simulink model "mc_pos"  (R2021a)
settings: Solver=FixedStepAuto  StartTime=0.0  StopTime=10.0  FixedStep=0.1  RelTol=1e-3
undefined symbols (not defined in the file): CONSTANTS_ONE_G, DiscIntNeverNeededParam, MPC_LAND_SPEED, MPC_SPOOLUP_TIME, MPC_THR_HOVER, MPC_THR_MAX, MPC_THR_MIN, MPC_TILTMAX_AIR, MPC_TILTMAX_LND, MPC_TKO_RAMP_T, MPC_VELD_LP, MPC_XY_P, MPC_XY_VEL_D_ACC, MPC_XY_VEL_I_ACC, MPC_XY_VEL_MAX, MPC_XY_VEL_P_ACC, MPC_Z_P, MPC_Z_VEL_D_ACC, MPC_Z_VEL_I_ACC, MPC_Z_VEL_MAX_DN, MPC_Z_VEL_MAX_UP, MPC_Z_VEL_P_ACC, PX4_TAKEOFF_STATUS, WV_EN
libraries: simulink x16, vrlib x2, sharedtransform x2, aerolibconvert2 x1
(part 2 of 3)

== system mc_pos/Position Controller/Position Control/addIfNotNan ==
  setpoint : Inport
  addition : Inport  Port=2
  AND : Logic  AllPortsSameDT=off  OutDataTypeStr=boolean
  IsFinite : RelationalOperator  Operator=isFinite  OutDataTypeStr=boolean  RndMeth=Simplest
  IsFinite1 : RelationalOperator  Operator=isFinite  OutDataTypeStr=boolean  RndMeth=Simplest
  IsFinite3 : RelationalOperator  Operator=isFinite  OutDataTypeStr=boolean  RndMeth=Simplest
  Sum : Sum  Inputs=++|
  Switch : Switch  Criteria=u2 ~= 0
  Switch1 : Switch  Criteria=u2 ~= 0
  addition1 : InportShadow  Port=2
  addition2 : InportShadow  Port=2
  setpoint1 : InportShadow
  setpoint2 : InportShadow
  sp_out : Outport
  wires:
  setpoint/1 -> IsFinite/1
  addition/1 -> IsFinite1/1
  IsFinite/1 -> AND/1
  IsFinite1/1 -> AND/2
  AND/1 -> Switch/2
  Sum/1 -> Switch/1
  setpoint1/1 -> Sum/2
  addition1/1 -> Sum/1
  Switch1/1 -> Switch/3
  setpoint2/1 -> IsFinite3/1, Switch1/1
  IsFinite3/1 -> Switch1/2
  addition2/1 -> Switch1/3
  Switch/1 -> sp_out/1

== system mc_pos/Position Controller/Position Control/addIfNotNan1 ==
  setpoint : Inport
  addition : Inport  Port=2
  AND : Logic  AllPortsSameDT=off  OutDataTypeStr=boolean
  IsFinite : RelationalOperator  Operator=isFinite  OutDataTypeStr=boolean  RndMeth=Simplest
  IsFinite1 : RelationalOperator  Operator=isFinite  OutDataTypeStr=boolean  RndMeth=Simplest
  IsFinite3 : RelationalOperator  Operator=isFinite  OutDataTypeStr=boolean  RndMeth=Simplest
  Sum : Sum  Inputs=++|
  Switch : Switch  Criteria=u2 ~= 0
  Switch1 : Switch  Criteria=u2 ~= 0
  addition1 : InportShadow  Port=2
  addition2 : InportShadow  Port=2
  setpoint1 : InportShadow
  setpoint2 : InportShadow
  sp_out : Outport
  wires:
  Switch/1 -> sp_out/1
  addition2/1 -> Switch1/3
  IsFinite3/1 -> Switch1/2
  setpoint2/1 -> Switch1/1, IsFinite3/1
  Switch1/1 -> Switch/3
  addition1/1 -> Sum/1
  setpoint1/1 -> Sum/2
  Sum/1 -> Switch/1
  AND/1 -> Switch/2
  IsFinite1/1 -> AND/2
  IsFinite/1 -> AND/1
  addition/1 -> IsFinite1/1
  setpoint/1 -> IsFinite/1

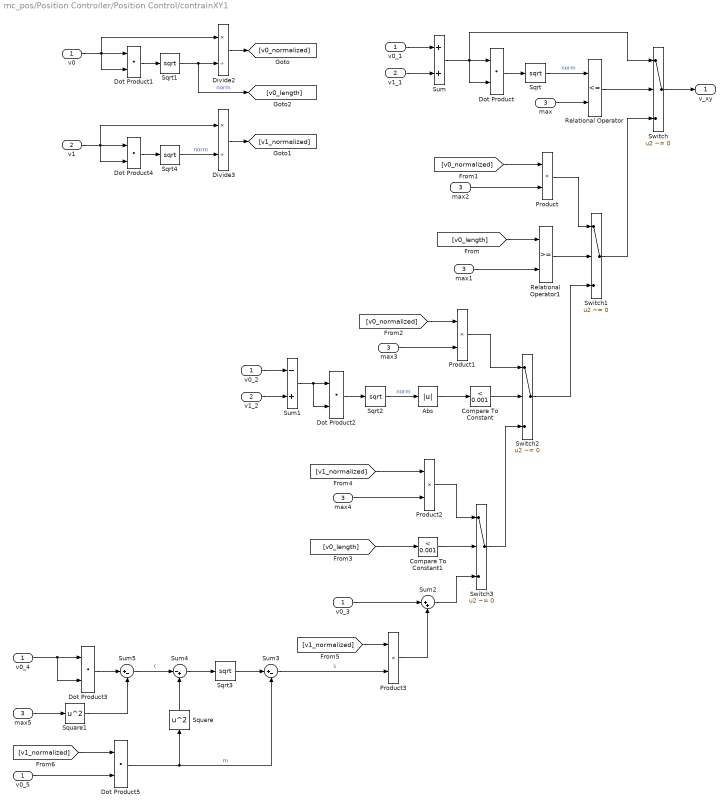
== system mc_pos/Position Controller/Position Control/contrainXY1 ==
  v0 : Inport
  v1 : Inport  Port=2
  max : Inport  Port=3
  Abs : Abs
  Compare To Constant : simulink/Logic and Bit Operations/Compare To Constant  relop=<  const=0.001  OutDataTypeStr=boolean
  Compare To Constant1 : simulink/Logic and Bit Operations/Compare To Constant  relop=<  const=0.001  OutDataTypeStr=boolean
  Divide2 : Product  Inputs=*/
  Divide3 : Product  Inputs=*/
  Dot Product{,1..5} (6 alike) : DotProduct  InputSameDT=on  OutDataTypeStr=Inherit: Inherit via internal rule
  Product{,1..3} (4 alike) : Product
  Relational Operator : RelationalOperator  Operator=<=  OutDataTypeStr=boolean  RndMeth=Simplest
  Relational Operator1 : RelationalOperator  OutDataTypeStr=boolean  RndMeth=Simplest
  Sqrt{,1..4} (5 alike) : Sqrt  SaturateOnIntegerOverflow=on
  Square : Math  Operator=square  SaturateOnIntegerOverflow=on
  Square1 : Math  Operator=square  SaturateOnIntegerOverflow=on
  Sum : Sum
  Sum1 : Sum  Inputs=-+
  Sum2 : Sum  Inputs=|++
  Sum3 : Sum  Inputs=|+-
  Sum4 : Sum  Inputs=|-+
  Sum5 : Sum  Inputs=|+-
  Switch{,1..3} (4 alike) : Switch  Criteria=u2 ~= 0
  max{1..5} (5 alike) : InportShadow  Port=3
  v0_{1..5} (5 alike) : InportShadow
  v1_1 : InportShadow  Port=2
  v1_2 : InportShadow  Port=2
  v_xy : Outport
  wires:
  v0_5/1 -> Dot Product5/2
  [v1_normalized] -> Dot Product5/1
  Square1/1 -> Sum5/2
  max5/1 -> Square1/1
  Dot Product3/1 -> Sum5/1
  v0_4/1 -> Dot Product3/1, Dot Product3/2
  Sum5/1 -> Sum4/1  "c"
  Square/1 -> Sum4/2
  Dot Product5/1 -> Sum3/2, Square/1  "m"
  Sum4/1 -> Sqrt3/1
  Sqrt3/1 -> Sum3/1
  Sum3/1 -> Product3/2  "s"
  [v1_normalized] -> Product3/1
  Product3/1 -> Sum2/2
  v0_3/1 -> Sum2/1
  Sum2/1 -> Switch3/3
  [v1_normalized] -> Product2/1
  max4/1 -> Product2/2
  Product2/1 -> Switch3/1
  [v0_length] -> Compare To Constant1/1
  Compare To Constant1/1 -> Switch3/2
  max3/1 -> Product1/2
  Product1/1 -> Switch2/1
  [v0_normalized] -> Product/1
  [v0_length] -> Relational Operator1/1
  Divide3/1 -> [v1_normalized]
  v1/1 -> Dot Product4/1, Dot Product4/2, Divide3/1
  Dot Product4/1 -> Sqrt4/1
  Sqrt4/1 -> Divide3/2  "norm"
  Divide2/1 -> [v0_normalized]
  Switch3/1 -> Switch2/3
  [v0_normalized] -> Product1/1
  v0_2/1 -> Sum1/1
  v1_2/1 -> Sum1/2
  Compare To Constant/1 -> Switch2/2
  Abs/1 -> Compare To Constant/1
  Sqrt2/1 -> Abs/1  "norm"
  Dot Product2/1 -> Sqrt2/1
  Sum1/1 -> Dot Product2/1, Dot Product2/2
  Switch2/1 -> Switch1/3
  Product/1 -> Switch1/1
  max2/1 -> Product/2
  Relational Operator1/1 -> Switch1/2
  max1/1 -> Relational Operator1/2
  Sqrt1/1 -> Divide2/2, [v0_length]  "norm"
  Dot Product1/1 -> Sqrt1/1
  v0/1 -> Dot Product1/1, Divide2/1, Dot Product1/2
  Switch1/1 -> Switch/3
  Switch/1 -> v_xy/1
  Relational Operator/1 -> Switch/2
  max/1 -> Relational Operator/2
  Sqrt/1 -> Relational Operator/1  "norm"
  Dot Product/1 -> Sqrt/1
  Sum/1 -> Dot Product/1, Dot Product/2, Switch/1
  v0_1/1 -> Sum/1
  v1_1/1 -> Sum/2

== system mc_pos/Position Controller/Velocity Control/I ==
  vel_error : Inport
  acc_sp : Inport  Port=2
  last_thr_sp : Inport  Port=3
  Bus Element In : Inport  Port=4  PortName=limit
  reset : Inport  Port=5
  Anti-Windup Calculate Velocity Error : Subsystem
  Constant : Constant  Value=[0 0 0]  OutDataTypeStr=single
  Discrete-Time Integrator : DiscreteIntegrator  ExternalReset=level  SampleTime=-1  SaturateOnIntegerOverflow=on  LimitOutput=on  UpperSaturationLimit=[inf inf CONSTANTS_ONE_G]  LowerSaturationLimit=-[inf inf CONSTANTS_ONE_G]  ICPrevOutput=DiscIntNeverNeededParam  ICPrevScaledInput=DiscIntNeverNeededParam
  Gain : Gain  Gain=[MPC_XY_VEL_I_ACC; MPC_XY_VEL_I_ACC; MPC_Z_VEL_I_ACC]
      settings: AttributesFormatString=%<Gain>
  addIfNotNan : Subsystem
  vel_init : Outport
  wires:
  Gain/1 -> Discrete-Time Integrator/1
  last_thr_sp/1 -> Anti-Windup Calculate Velocity Error/3(last_thr_sp)
  Bus Element In/1 -> Anti-Windup Calculate Velocity Error/4(limit)
  vel_error/1 -> Anti-Windup Calculate Velocity Error/1(vel_error)
  acc_sp/1 -> Anti-Windup Calculate Velocity Error/2(acc_sp)
  Discrete-Time Integrator/1 -> vel_init/1
  reset/1 -> Discrete-Time Integrator/2
  Anti-Windup Calculate Velocity Error/1(vel_error_out) -> addIfNotNan/1(setpoint)
  Constant/1 -> addIfNotNan/2(addition)
  addIfNotNan/1(sp_out) -> Gain/1

== system mc_pos/Position Controller/Velocity Control/addIfNotNan ==
  setpoint : Inport
  addition : Inport  Port=2
  AND : Logic  AllPortsSameDT=off  OutDataTypeStr=boolean
  IsFinite : RelationalOperator  Operator=isFinite  OutDataTypeStr=boolean  RndMeth=Simplest
  IsFinite1 : RelationalOperator  Operator=isFinite  OutDataTypeStr=boolean  RndMeth=Simplest
  IsFinite3 : RelationalOperator  Operator=isFinite  OutDataTypeStr=boolean  RndMeth=Simplest
  Sum : Sum  Inputs=++|
  Switch : Switch  Criteria=u2 ~= 0
  Switch1 : Switch  Criteria=u2 ~= 0
  addition1 : InportShadow  Port=2
  addition2 : InportShadow  Port=2
  setpoint1 : InportShadow
  setpoint2 : InportShadow
  sp_out : Outport
  wires:
  setpoint/1 -> IsFinite/1
  addition/1 -> IsFinite1/1
  IsFinite/1 -> AND/1
  IsFinite1/1 -> AND/2
  AND/1 -> Switch/2
  Sum/1 -> Switch/1
  setpoint1/1 -> Sum/2
  addition1/1 -> Sum/1
  Switch1/1 -> Switch/3
  setpoint2/1 -> IsFinite3/1, Switch1/1
  IsFinite3/1 -> Switch1/2
  addition2/1 -> Switch1/3
  Switch/1 -> sp_out/1

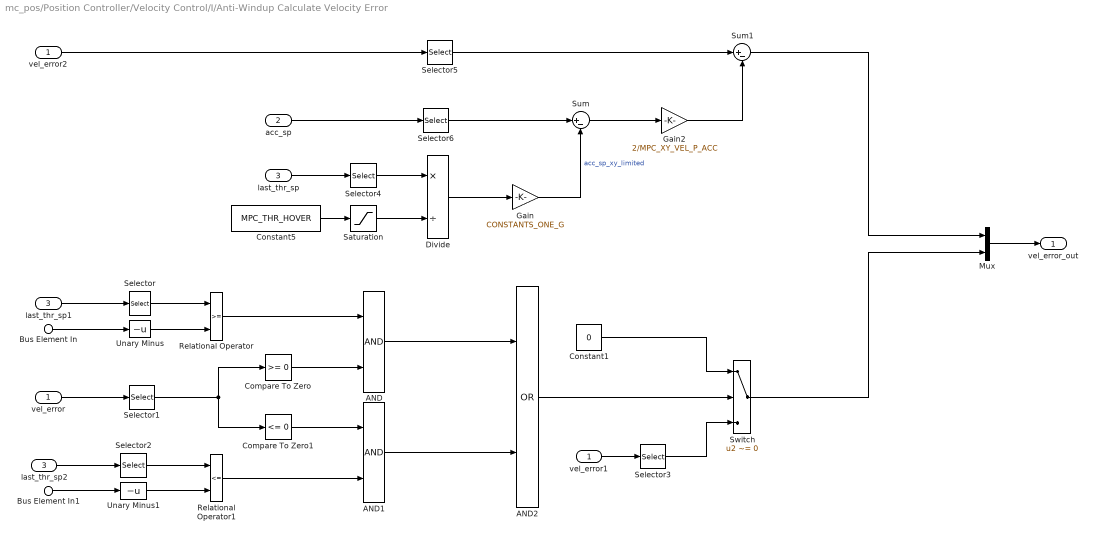
== system mc_pos/Position Controller/Velocity Control/I/Anti-Windup Calculate Velocity Error ==
  vel_error : Inport
  acc_sp : Inport  Port=2
  last_thr_sp : Inport  Port=3
  Bus Element In : Inport  Port=4  PortName=limit  Element=lim_thr_min
  Bus Element In1 : Inport  Port=4  PortName=limit  Element=lim_thr_max
  AND : Logic  AllPortsSameDT=off  OutDataTypeStr=boolean
  AND1 : Logic  AllPortsSameDT=off  OutDataTypeStr=boolean
  AND2 : Logic  Operator=OR  AllPortsSameDT=off  OutDataTypeStr=boolean
  Compare To Zero : simulink/Logic and Bit Operations/Compare To Zero  relop=>=  OutDataTypeStr=boolean
  Compare To Zero1 : simulink/Logic and Bit Operations/Compare To Zero  relop=<=  OutDataTypeStr=boolean
  Constant1 : Constant  Value=0  OutDataTypeStr=single
  Constant5 : Constant  Value=MPC_THR_HOVER  OutDataTypeStr=single
  Divide : Product  Inputs=*/
  Gain : Gain  Gain=CONSTANTS_ONE_G
      settings: AttributesFormatString=%<Gain>
  Gain2 : Gain  Gain=2/MPC_XY_VEL_P_ACC
      settings: AttributesFormatString=%<Gain>
  Mux : Mux  Inputs=2
  Relational Operator : RelationalOperator  OutDataTypeStr=boolean  RndMeth=Simplest
  Relational Operator1 : RelationalOperator  Operator=<=  OutDataTypeStr=boolean  RndMeth=Simplest
  Saturation : Saturate  UpperLimit=0.9  LowerLimit=0.1
      settings: AttributesFormatString=[%<LowerLimit>, %<UpperLimit>]
  Selector{,1..3} (4 alike) : Selector  InputPortWidth=3  IndexOptions=Index vector (dialog)  Indices=3  OutputSizes=1
  Selector4 : Selector  InputPortWidth=3  IndexOptions=Index vector (dialog)  Indices=[1 2]  OutputSizes=1
  Selector5 : Selector  InputPortWidth=3  IndexOptions=Index vector (dialog)  Indices=[1 2]  OutputSizes=1
  Selector6 : Selector  InputPortWidth=3  IndexOptions=Index vector (dialog)  Indices=[1 2]  OutputSizes=1
  Sum : Sum  Inputs=|+-
  Sum1 : Sum  Inputs=|+-
  Switch : Switch  Criteria=u2 ~= 0
  Unary Minus : UnaryMinus
  Unary Minus1 : UnaryMinus
  last_thr_sp1 : InportShadow  Port=3
  last_thr_sp2 : InportShadow  Port=3
  vel_error1 : InportShadow
  vel_error2 : InportShadow
  vel_error_out : Outport
  wires:
  Selector1/1 -> Compare To Zero/1, Compare To Zero1/1
  Compare To Zero1/1 -> AND1/1
  Unary Minus/1 -> Relational Operator/2
  Selector/1 -> Relational Operator/1
  AND2/1 -> Switch/2
  Selector2/1 -> Relational Operator1/1
  Unary Minus1/1 -> Relational Operator1/2
  Constant1/1 -> Switch/1
  Relational Operator/1 -> AND/1
  AND1/1 -> AND2/2
  Selector3/1 -> Switch/3
  Compare To Zero/1 -> AND/2
  Relational Operator1/1 -> AND1/2
  vel_error1/1 -> Selector3/1
  AND/1 -> AND2/1
  Bus Element In/1 -> Unary Minus/1
  Bus Element In1/1 -> Unary Minus1/1
  last_thr_sp1/1 -> Selector/1
  last_thr_sp2/1 -> Selector2/1
  vel_error/1 -> Selector1/1
  Switch/1 -> Mux/2
  last_thr_sp/1 -> Selector4/1
  Selector4/1 -> Divide/1
  Divide/1 -> Gain/1
  vel_error2/1 -> Selector5/1
  acc_sp/1 -> Selector6/1
  Selector6/1 -> Sum/1
  Sum1/1 -> Mux/1
  Constant5/1 -> Saturation/1
  Gain/1 -> Sum/2  "acc_sp_xy_limited"
  Saturation/1 -> Divide/2
  Sum/1 -> Gain2/1
  Selector5/1 -> Sum1/1
  Gain2/1 -> Sum1/2
  Mux/1 -> vel_error_out/1

== system mc_pos/Position Controller/Velocity Control/I/addIfNotNan ==
  setpoint : Inport
  addition : Inport  Port=2
  AND : Logic  AllPortsSameDT=off  OutDataTypeStr=boolean
  IsFinite : RelationalOperator  Operator=isFinite  OutDataTypeStr=boolean  RndMeth=Simplest
  IsFinite1 : RelationalOperator  Operator=isFinite  OutDataTypeStr=boolean  RndMeth=Simplest
  IsFinite3 : RelationalOperator  Operator=isFinite  OutDataTypeStr=boolean  RndMeth=Simplest
  Sum : Sum  Inputs=++|
  Switch : Switch  Criteria=u2 ~= 0
  Switch1 : Switch  Criteria=u2 ~= 0
  addition1 : InportShadow  Port=2
  addition2 : InportShadow  Port=2
  setpoint1 : InportShadow
  setpoint2 : InportShadow
  sp_out : Outport
  wires:
  setpoint/1 -> IsFinite/1
  addition/1 -> IsFinite1/1
  IsFinite/1 -> AND/1
  IsFinite1/1 -> AND/2
  AND/1 -> Switch/2
  Sum/1 -> Switch/1
  setpoint1/1 -> Sum/2
  addition1/1 -> Sum/1
  Switch1/1 -> Switch/3
  setpoint2/1 -> IsFinite3/1, Switch1/1
  IsFinite3/1 -> Switch1/2
  addition2/1 -> Switch1/3
  Switch/1 -> sp_out/1

== stateflow chart mc_pos/Handle Smooth Takeoff ==
  state UpdateTakeoffState
    state result = tilt_limit_slew_rate_update(input) [function]
    state Disarmed
      en:
      takeoff_state = uint8(PX4_TAKEOFF_STATUS.TAKEOFF_STATE_DISARMED);
      en,du:
      % 加速度限幅，没起飞前z轴的accel setpoint设为nan，取消在跑道上加速度的前馈
      setpoint_output.acceleration(3) = single(nan);
      % setpoint限幅，起飞前禁止任何的校正
      setpoint_output = UpdateTakeoffState.reset_setpoint_to_nan(setpoint);
      % 重置速度积分
      vel_reset_integral = true;
      % 倾角限幅
      limit.lim_tilt = UpdateTakeoffState.tilt_limit_slew_rate_update(MPC_TILTMAX_LND);
      % 向上速度限幅
      speed_up = -CONSTANTS_ONE_G / max(MPC_Z_VEL_P_ACC, 0.01);
      limit.lim_vel_up = min(speed_up, MPC_Z_VEL_MAX_DN);
      % 向下速度限幅
      speed_down = constraints.speed_down;
      if (~isfinite(speed_down))
      speed_down = single(MPC_Z_VEL_MAX_DN);
      end
      limit.lim_vel_down = constrain(speed_down, 0.0, MPC_Z_VEL_MAX_DN);
      % 水平速度限幅
      speed_horizontal = constraints.speed_xy;
      if (~isfinite(speed_horizontal))
      speed_horizontal = single(MPC_XY_VEL_MAX);
      end
      limit.lim_vel_horizontal = constrain(speed_horizontal, 0.0, MPC_XY_VEL_MAX);
      % 油门限幅
      limit.lim_thr_min = 1e-5;
      limit.lim_thr_max = MPC_THR_MAX;
    state Spool_Up
      en:
      takeoff_state = uint8(PX4_TAKEOFF_STATUS.TAKEOFF_STATE_SPOOLUP);
      en,du:
      % 加速度限幅，没起飞前z轴的accel setpoint设为nan，取消在跑道上加速度的前馈
      setpoint_output.acceleration(3) = single(nan);
      % setpoint限幅，起飞前禁止任何的校正
      setpoint_output = UpdateTakeoffState.reset_setpoint_to_nan(setpoint);
      % 重置速度积分
      vel_reset_integral = true;
      % 倾角限幅
      limit.lim_tilt = UpdateTakeoffState.tilt_limit_slew_rate_update(MPC_TILTMAX_LND);
      % 向上速度限幅
      speed_up = -CONSTANTS_ONE_G / max(MPC_Z_VEL_P_ACC, 0.01);
      limit.lim_vel_up = min(speed_up, MPC_Z_VEL_MAX_DN);
      % 向下速度限幅
      speed_down = constraints.speed_down;
      if (~isfinite(speed_down))
      speed_down = single(MPC_Z_VEL_MAX_DN);
      end
      limit.lim_vel_down = constrain(speed_down, 0.0, MPC_Z_VEL_MAX_DN);
      % 水平速度限幅
      speed_horizontal = constraints.speed_xy;
      if (~isfinite(speed_horizontal))
      speed_horizontal = single(MPC_XY_VEL_MAX);
      end
      limit.lim_vel_horizontal = constrain(speed_horizontal, 0.0, MPC_XY_VEL_MAX);
      % 油门限幅
      limit.lim_thr_min = 1e-5;
      limit.lim_thr_max = MPC_THR_MAX;
    state Ready_Takeoff
      en:
      takeoff_state = uint8(PX4_TAKEOFF_STATUS.TAKEOFF_STATE_READY_FOR_TAKEOFF);
      en,du:
      % 加速度限幅，没起飞前z轴的accel setpoint设为nan，取消在跑道上加速度的前馈
      setpoint_output.acceleration(3) = single(nan);
      % setpoint限幅，起飞前禁止任何的校正
      setpoint_output = UpdateTakeoffState.reset_setpoint_to_nan(setpoint);
      % 重置速度积分
      vel_reset_integral = true;
      % 倾角限幅
      limit.lim_tilt = UpdateTakeoffState.tilt_limit_slew_rate_update(MPC_TILTMAX_LND);
      % 向上速度限幅
      speed_up = -CONSTANTS_ONE_G / max(MPC_Z_VEL_P_ACC, 0.01);
      limit.lim_vel_up = min(speed_up, MPC_Z_VEL_MAX_DN);
      % 向下速度限幅
      speed_down = constraints.speed_down;
      if (~isfinite(speed_down))
      speed_down = single(MPC_Z_VEL_MAX_DN);
      end
      limit.lim_vel_down = constrain(speed_down, 0.0, MPC_Z_VEL_MAX_DN);
      % 水平速度限幅
      speed_horizontal = constraints.speed_xy;
      if (~isfinite(speed_horizontal))
      speed_horizontal = single(MPC_XY_VEL_MAX);
      end
      limit.lim_vel_horizontal = constrain(speed_horizontal, 0.0, MPC_XY_VEL_MAX);
      % 油门限幅
      limit.lim_thr_min = 1e-5;
      limit.lim_thr_max = MPC_THR_MAX;
    state Ramp_Up
      en:
      takeoff_state = uint8(PX4_TAKEOFF_STATUS.TAKEOFF_STATE_RAMPUP);
      en,du:
      setpoint_output = setpoint;
      % 加速度限幅，没起飞前z轴的accel setpoint设为nan，取消在跑道上加速度的前馈
      setpoint_output.acceleration(3) = single(nan);
      % 允许速度积分
      vel_reset_integral = false;
      % 倾角限幅
      limit.lim_tilt = UpdateTakeoffState.tilt_limit_slew_rate_update(MPC_TILTMAX_LND);
      % 向上速度限幅
      speed_up = constraints.speed_up;
      if (~isfinite(constraints.speed_up))
      speed_up = single(MPC_Z_VEL_MAX_UP);
      end
      takeoff_ramp_progress = elapsed(sec) / MPC_TKO_RAMP_T;
      takeoff_ramp_vz_init = -CONSTANTS_ONE_G / max(MPC_Z_VEL_P_ACC, 0.01);
      if (takeoff_ramp_progress < 1.0)
      limit.lim_vel_up = takeoff_ramp_vz_init + takeoff_ramp_progress * (speed_up - takeoff_ramp_vz_init);
      end
      % 向下速度限幅
      speed_down = constraints.speed_down;
      if (~isfinite(speed_down))
      speed_down = single(MPC_Z_VEL_MAX_DN);
      end
      limit.lim_vel_down = constrain(speed_down, 0.0, MPC_Z_VEL_MAX_DN);
      % 水平速度限幅
      speed_horizontal = constraints.speed_xy;
      if (~isfinite(speed_horizontal))
      speed_horizontal = single(MPC_XY_VEL_MAX);
      end
      limit.lim_vel_horizontal = constrain(speed_horizontal, 0.0, MPC_XY_VEL_MAX);
      % 油门限幅
      limit.lim_thr_min = 1e-5;
      limit.lim_thr_max = MPC_THR_MAX;
    state Flight
      en:
      takeoff_state = uint8(PX4_TAKEOFF_STATUS.TAKEOFF_STATE_FLIGHT);
      en,du:
      setpoint_output = setpoint;
      % 倾角限幅
      limit.lim_tilt = UpdateTakeoffState.tilt_limit_slew_rate_update(MPC_TILTMAX_AIR);
      % 允许速度积分
      vel_reset_integral = false;
      % 向上速度限幅
      speed_up = constraints.speed_up;
      if (~isfinite(constraints.speed_up))
      speed_up = single(MPC_Z_VEL_MAX_UP);
      end
      limit.lim_vel_up = speed_up;
      % 向下速度限幅
      speed_down = constraints.speed_down;
      if (~isfinite(speed_down))
      speed_down = single(MPC_Z_VEL_MAX_DN);
      end
      limit.lim_vel_down = constrain(speed_down, 0.0, MPC_Z_VEL_MAX_DN);
      % 水平速度限幅
      speed_horizontal = constraints.speed_xy;
      if (~isfinite(speed_horizontal))
      speed_horizontal = single(MPC_XY_VEL_MAX);
      end
      limit.lim_vel_horizontal = constrain(speed_horizontal, 0.0, MPC_XY_VEL_MAX);
      % 油门限幅
      limit.lim_thr_min = max(MPC_THR_MIN, 1e-5);
      limit.lim_thr_max = MPC_THR_MAX;
    state Flying_GroundContact
      en,du:
      % setpoint限幅，起飞前禁止任何的校正
      setpoint_output = UpdateTakeoffState.reset_setpoint_to_nan(setpoint);
      % 重置速度积分
      vel_reset_integral = true;
      % 倾角限幅
      limit.lim_tilt = UpdateTakeoffState.tilt_limit_slew_rate_update(MPC_TILTMAX_LND);
      % 向上速度限幅
      speed_up = -CONSTANTS_ONE_G / max(MPC_Z_VEL_P_ACC, 0.01);
      limit.lim_vel_up = min(speed_up, MPC_Z_VEL_MAX_DN);
      % 向下速度限幅
      speed_down = constraints.speed_down;
      if (~isfinite(speed_down))
      speed_down = single(MPC_Z_VEL_MAX_DN);
      end
      limit.lim_vel_down = constrain(speed_down, 0.0, MPC_Z_VEL_MAX_DN);
      % 水平速度限幅
      speed_horizontal = constraints.speed_xy;
      if (~isfinite(speed_horizontal))
      speed_horizontal = single(MPC_XY_VEL_MAX);
      end
      limit.lim_vel_horizontal = constrain(speed_horizontal, 0.0, MPC_XY_VEL_MAX);
      % 油门限幅
      limit.lim_thr_min = 1e-5;
      limit.lim_thr_max = MPC_THR_MAX;
    UpdateTakeoffState -> Flight [order 2] : [control_mode.flag_armed && skip_takeoff]
    (default) -> Disarmed
    Ready_Takeoff -> Ramp_Up : [constraints.want_takeoff]
    Disarmed -> Spool_Up : [control_mode.flag_armed]
    Ramp_Up -> Flight : [takeoff_ramp_progress >= 1.0]
    Spool_Up -> Ready_Takeoff : [after(MPC_SPOOLUP_TIME, sec)]
    Flight -> Flying_GroundContact [order 1] : [land_detected.ground_contact]
    UpdateTakeoffState -> Disarmed [order 1] : [~control_mode.flag_armed]
    (junction 105) -> Ready_Takeoff
    Flight -> (junction 106) [order 2]
    Flying_GroundContact -> (junction 113)
    (junction 106) -> (junction 105) : [land_detected.landed]
    (junction 113) -> (junction 106) : [land_detected.landed]
  data: result function_output; input function_input; input function_input double size=1; result function_output; speed_up local single size=1; speed_down local single size=1; speed_horizontal local single size=1; constraints input Bus: px4_vehicle_constraints; setpoint_output output Bus: px4_vehicle_local_position_setpoint; control_mode input Bus: px4_vehicle_control_mode; land_detected input Bus: px4_vehicle_land_detected; skip_takeoff input; setpoint input Bus: px4_vehicle_local_position_setpoint; takeoff_ramp_progress local; vel_reset_integral output boolean; limit output Bus: px4_mc_pos_limit; MPC_TILTMAX_AIR parameter; MPC_TILTMAX_LND parameter; MPC_Z_VEL_MAX_DN parameter; MPC_XY_VEL_MAX parameter; MPC_THR_MAX parameter; MPC_THR_MIN parameter; takeoff_ramp_vz_init local; CONSTANTS_ONE_G parameter; MPC_Z_VEL_P_ACC parameter; MPC_Z_VEL_MAX_UP parameter; MPC_TKO_RAMP_T parameter; MPC_SPOOLUP_TIME parameter single size=1; takeoff_state output uint8
  function result = reset_setpoint_to_nan(input):
    | function result = reset_setpoint_to_nan(input)
    | 
    | result = input;
    | 
    | result.x = single(nan);
    | result.y = single(nan);
    | result.z = single(nan);
    | 
    | result.vx = single(nan);
    | result.vy = single(nan);
    | result.vz = single(nan);
    | 
    | result.yaw = single(nan);
    | result.yawspeed = single(nan);
    | 
    | % High downwards acceleration to make sure there's no thrust
    | result.acceleration = single([0.0; 0.0; 100]);
    | 
    | result.thrust = single([nan; nan; nan]);
    | 
    | end

== matlab function mc_pos/Generate Attitude Setpoint/Publish Takeoff Status/MATLAB Function ==
  data: x input; result output; y input; eps_value input
function result = isEqual(x, y, eps_value)

result = (abs(x - y) <= eps_value) || (isnan(x) && isnan(y)) || (isinf(x) && isinf(y) && isnan(x - y));

end

== matlab function mc_pos/Position Controller/Position Control/MATLAB Function ==
  data: y output; v0 input; v1 input; max input
function y = constrainXY(v0, v1, max)

if (norm(v0 + v1) <= max)
    % vector does not exceed maximum magnitude
    y = v0 + v1;
elseif (norm(v0) >= max)
    % the magnitude along v0, which has priority, already exceeds maximum.
    y = v0 / norm(v0) * max;
elseif (abs(norm(v1 - v0)) < 0.001)
    % the two vectors are equal
    y =  v0 /norm(v0) * max;
elseif (norm(v0) < 0.001)
    % the first vector is 0.
    y =  v1 / norm(v1) * max;
else
    % vf = final vector with ||vf|| <= max
    % s = scaling factor
    % u1 = unit of v1
    % vf = v0 + v1 = v0 + s * u1
    % constraint: ||vf|| <= max
    %
    % solve for s: ||vf|| = ||v0 + s * u1|| <= max
    %
    % Derivation:
    % For simplicity, replace v0 -> v, u1 -> u
    % 				   		   v0(0/1/2) -> v0/1/2
    % 				   		   u1(0/1/2) -> u0/1/2
    %
    % ||v + s * u||^2 = (v0+s*u0)^2+(v1+s*u1)^2+(v2+s*u2)^2 = max^2
    % v0^2+2*s*u0*v0+s^2*u0^2 + v1^2+2*s*u1*v1+s^2*u1^2 + v2^2+2*s*u2*v2+s^2*u2^2 = max^2
    % s^2*(u0^2+u1^2+u2^2) + s*2*(u0*v0+u1*v1+u2*v2) + (v0^2+v1^2+v2^2-max^2) = 0
    %
    % quadratic equation:
    % -> s^2*a + s*b + c = 0 with solution: s1/2 = (-b +- sqrt(b^2 - 4*a*c))/(2*a)
    %
    % b = 2 * u.dot(v)
    % a = 1 (because u is normalized)
    % c = (v0^2+v1^2+v2^2-max^2) = -max^2 + ||v||^2
    %
    % sqrt(b^2 - 4*a*c) =
    % 		sqrt(4*u.dot(v)^2 - 4*(||v||^2 - max^2)) = 2*sqrt(u.dot(v)^2 +- (||v||^2 -max^2))
    %
    % s1/2 = ( -2*u.dot(v) +- 2*sqrt(u.dot(v)^2 - (||v||^2 -max^2)) / 2
    %      =  -u.dot(v) +- sqrt(u.dot(v)^2 - (||v||^2 -max^2))
    % m = u.dot(v)
    % s = -m + sqrt(m^2 - c)
    %
    %
    %
    % notes:
    % 	- s (=scaling factor) needs to be positive
    % 	- (max - ||v||) always larger than zero, otherwise it never entered this if-statement
    u1 = v1 / norm(v1);
    m = dot(u1, v0);
    c = dot(v0, v0) - max * max;
    s = -m + sqrt(m * m - c);
    y =  v0 + u1 * s;
end

end
